simulink model "scale"  (Simulink 3.00)
settings: Solver=ode45  StartTime=0.0  StopTime=10.0  RelTol=1e-3
settings Model: LastModifiedBy=campa

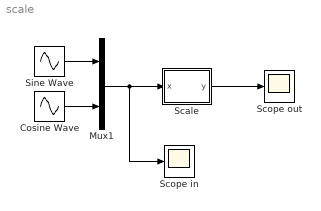
== system scale ==
  Cosine Wave : Sin  Amplitude=1  Frequency=1  Phase=pi/2  SampleTime=0
  Mux1 : Mux  Inputs=2
  Scale : Subsystem  mask(Scale){xmin=[-2 -1], xmax=[2 1], ymin=[0 -5], ymax=[6 7], r=on}
      mask prompts: xmin "x min"; xmax "x max"; ymin "y min"; ymax "y max"; r "Reshape parameters as 1D vectors"
      mask help:
      | Scales the input vector x, ranging from xmin to xmax,
      |    to an output vector y, ranging from ymin to ymax.
      |    Uncheck the checkbox to scale matrices instead of vectors.
      mask init:
      | if r,
      | 	xmin=xmin(:);
      | 	xmax=xmax(:);
      | 	ymin=ymin(:);
      | 	ymax=ymax(:);
      | end
      mask Help:
      | Scales the input vector x, ranging from xmin to xmax,
      |    to an output vector y, ranging from ymin to ymax.
      |    Uncheck the checkbox to scale matrices instead of vectors.
      |    <br><br>
      |    The checkbox has been included because sometimes it is simpler to    enter parameters as matrices and then let the block reshape them to
      |    vectors internally.
      |    <br>
      |    On the other hand parameters must have the same dimensions of the input       and output signals, so if one wants to scale matrices, the parameter must
      |    be matrices and should not be reshaped, so the checkbox has to be
      |    unchecked in that case.
      |    <br><br>
      |    Matlab 5.3 does not support matrices and rechapes parameters to matrices
      |    anyway, so in that version the checkbox has no influence.
  Scope in : Scope
      settings: TimeRange=auto  YMin=-5  YMax=5  SaveToWorkspace=off  SaveName=ScopeData
  Scope out : Scope
      settings: TimeRange=10  YMin=-5  YMax=10  SaveToWorkspace=off  SaveName=ScopeData
  Sine Wave : Sin  Amplitude=2  Frequency=1  Phase=0  SampleTime=0
  wires:
  Scale/1(y) -> Scope out/1
  Sine Wave/1 -> Mux1/1
  Cosine Wave/1 -> Mux1/2
  Mux1/1 -> Scale/1(x), Scope in/1

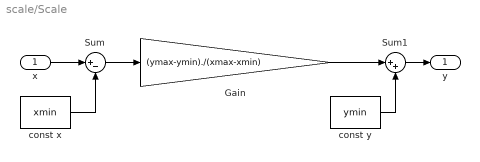
== system scale/Scale ==
  x : Inport  Port=1  PortWidth=-1  SampleTime=-1  DataType=auto
      settings: SignalType=auto
  Gain : Gain  Gain=(ymax-ymin)./(xmax-xmin)  SaturateOnIntegerOverflow=on
  Sum : Sum  Inputs=|+-  SaturateOnIntegerOverflow=on
  Sum1 : Sum  Inputs=|++  SaturateOnIntegerOverflow=on
  const x : Constant  Value=xmin
  const y : Constant  Value=ymin
  y : Outport  Port=1
  wires:
  x/1 -> Sum/1
  Sum/1 -> Gain/1
  const x/1 -> Sum/2
  Gain/1 -> Sum1/1
  Sum1/1 -> y/1
  const y/1 -> Sum1/2
